simulink library "simetran"  (R2024b)
settings: Solver=VariableStepAuto  StartTime=0.0  StopTime=10.0  RelTol=1e-3
undefined symbols (not defined in the file): Csnu, gcbh, h, ResistanceM, Rsnu, Rt4, sps_rtmsupport, Ti, Ts, Z, Zm
libraries: fl_lib x81, nesl_utility x48, ee_lib x23
(part 1 of 3)
settings Model: Creator=Kyle  LastModifiedBy=CD8435

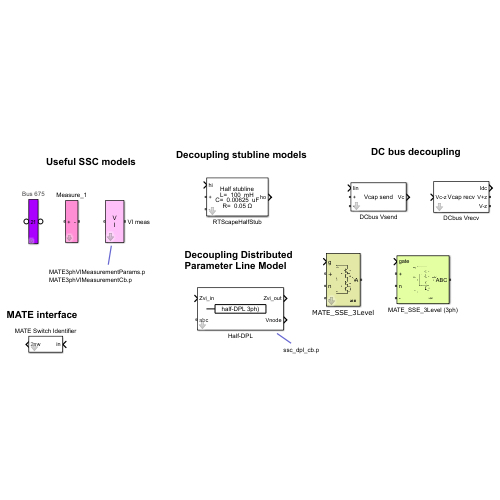
[thumbnail: Simulink's stored preview of the top-level diagram]
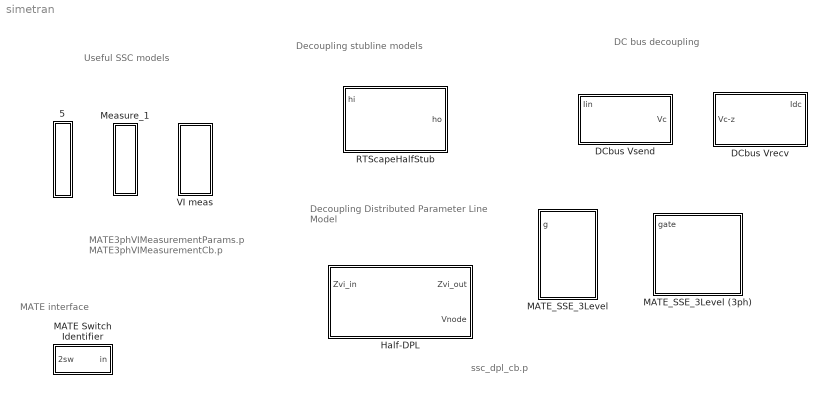
== system simetran ==
  note: ssc_dpl_cb.p
  note: MATE3phVIMeasurementParams.p
      | MATE3phVIMeasurementCb.p
  note: Decoupling stubline models
  note: Useful SSC models
  note: MATE interface
  note: DC bus decoupling
  note: Decoupling Distributed
      | Parameter Line Model
  5 : Subsystem  mask(Simscape Electrical Bus Numbering){bn=675}
      mask prompts: bn "Bus number"
      mask help: This block is a simple passthrough
      settings: AttributesFormatString=Bus %<bn>
  DCbus Vrecv : Subsystem  mask(DC Bus decoupling (Receiving-V)){Ts=Ts}
      mask prompts: Ts "Sample time (s)"
      mask help: This block is used to create a delay in DC-busses..
      mask Display: disp('Vcap recv')
  DCbus Vsend : Subsystem  mask(DC Bus decoupling (Sending-V)){Ts=Ts}
      mask prompts: Ts "Sample time (s)"
      mask help: This block is used to create a delay in DC-busses.
      mask Display: disp('Vcap send')
  Half-DPL : Subsystem  mask(Simscape 3-phase Distributed Parameters Line){Phases=3, Frequency=60, Resistance=[0.01273*2 0.3864], Inductance=[0.9337e-3  4.1264e-3], Capacitance=[12.74e-9 7.751e-9], Length=75, Ts=Ts}
      mask prompts: Phases "Number of phases N"; Frequency "Frequency used for R L C specification (Hz)"; Resistance "Resistance per unit length (Ohms/km)   [N*N matrix] or [R1 R0 R0m]"; Inductance "Inductance per unit length (H/km) [N*N matrix ] or [L1 L0 L0m]"; Capacitance "Capacitance per unit length (F/km) [N*N matrix] or [C1 C0 C0m]"; Length "Line length (km)"; Ts "Sample time (s)"
      mask help:
      | Implements a 3-phases distributed parameter line (DPL) model.
      |
      | One can either specify complete [NxN] matrices or simply enter sequence parameters vectors: the  positive and zero sequence parameters for a two-phase or  three-phase transposed  line, plus the mutual zero-sequence for a  six-phase transposed  line  (2 coupled 3-phase lines).
      |
      | This DPL model allows the decoupling of computational tasks at each line ends.
      mask init:
      | % Get current block
      | currentBlock = gcb;
      | 
      | % Get electric variables
      | [Zm,R,v,Ti,to,Rt4,h,Zimp,Zmat,Yphase,ResistanceM] = ssc_dpl_cb(gcb,'funcky balls', Phases, Frequency, Resistance, Inductance, Capacitance, Length);
      | 
      | delay=floor(to/Ts);
      | remd=rem(to,Ts)/Ts;
      | 
      | mess=['SimScape \n\n\n' ' DPL 3-ph'];
      mask TypeOptions Phases: 1 | 2 | 3 | 4 | 5 | 6 | 8 | 9 | 10 | 12
      mask Display:
      | plot(0,0,100,100,[20,20,80,80,80,80,20,20,10],[50,40,40,50,50,61,61,50,50])
      | disp('half-DPL 3ph)')
      | %disp(mess)
  MATE Switch Identifier : Subsystem  mask(MATE Switch Identifier){bn=Circuit BreakerEXP, bns=Circuit BreakerEXP, rsw=on, tagro=[]}
      mask prompts: bn "Switch block name (no ' ')"; bns "saved blockname"; rsw "Reverse switch logic"; tagro "Goto Tag (read only)"
      mask help: This block is used to identify switch signals for MATE optimization
      mask Callback bn:
      | this=gcb;
      | bns_x=get_param(this,'bns');
      | bn_x=get_param(this,'bn');
      | if ~isequal(bns_x, bn_x)
      |     set_param(this,'bns',bn_x);
      |     str=tempname;
      |     str=strrep(str(end-20:end),'_','x');
      |     str=['a' str];
      |     set_param([this '/Goto'],'Gototag',str);
      | end
      | gt=get_param([this '/Goto'],'GotoTag');
      | set_param([this],'tagro',gt);
      mask DialogControl Control2 Prompt: Note: Simscape electric breaker in open (OFF) when gate=1)
      mask DialogControl Control3 Prompt: Note: by using revert logic, it becomes like SPS breaker
  MATE_SSE_3Level : Subsystem  DialogController=POWERSYS.PowerSysDialog  mask(MATE 3-level NPC inverter){Arms=1, SnubberResistance=Rsnu, SnubberCapacitance=Csnu, Device=IGBT / Diodes, Ron=1e-3, Vf=1, ihiz=999}
      mask prompts: Arms "Number of bridge arms:"; SnubberResistance "Snubber resistance Rs (Ohms)"; SnubberCapacitance "Snubber capacitance Cs (F)"; Device "Power Electronic device (IGBT, GTO,MOSFET are equivalent)"; Ron "Internal resistance Ron (Ohms)"; Vf "Forward Device voltage  (V)"; ihiz "High Impedance current tolerance"
      mask help:
      | MATE Three-Level Bridge
      |
      | This model implements a 3-level NPC inverter using a surrogate circuit.
      | The surrogate circuit has only 3 switches and associated RC snubber.
      | The 3 switches connects the output phase connection A to each of inputs of inverter(V+, N, V-) and are controlled using an algorithm that mimics the behavior of real 3-level NPC inverters.
      |
      | Parameters:
      |
      | Snubber resistance Rs (Ohms): Resistance of the RC-snubber.
      | Snubber capacitance Cs (F): Capacitance of the RC snubber.
      | Internal resistance Ron (Ohms): Conduction resistance of all switches.
      |
      | gate signal (size 4). Drive the 4 IGBTs from the + rail to neutral rail, to the - rail in this order.
      mask init:
      | X.p1= [39 39 23.8000];
      |     X.p2= [44 56 49.6000 56 52.8000 56 61 61];
      |     X.p3= [44 44 44 61 61];
      |     X.p4= [75 67 83 75 67 83 75 75];
      |     X.p5= [61 75 75];
      |     X.p6= [75 75 61];
      |     X.p7= 0;
      | 
      |     Y.p1= [71 28 28];
      |     Y.p2= [  39.2000   33.6000   32.8000   33.6000   40.8000   33.6000  30.0000   12.4000];
      |     Y.p3= [28 71 60 66.4000 90];
      |     Y.p4= [54 42 42 54 54 54 54 66];
      |     Y.p5= [24 24 42];
      |     Y.p6= [66 76 76];
      |     Y.p7= 0;
      mask TypeOptions Arms: 1
      mask TypeOptions Device: IGBT / Diodes
  MATE_SSE_3Level (3ph) : Subsystem
  Measure_1 : Subsystem  DialogController=POWERSYS.PowerSysDialog  StartFcn=sps_rtmsupport('StartFcn',gcbh);  StopFcn=sps_rtmsupport('StopFcn',gcbh);  mask(Three-Phase Measurement){Va=Vabc_633_ssc, Ia=Iabc_633_ssc}
      mask prompts: Va "Voltage signal label  (use a From block to collect this signal)"; Ia "Current signal label  (use a From block to collect this signal)"
      mask help:
      | Ideal three-phase voltage and current measurements.
      |
      | The block outputs the voltages and currents in volts and amperes at the corresponding From blocks
      mask init:
      | bloc = gcb;
      | 
      | Vtag=get_param(bloc,'Va');
      | Itag=get_param(bloc,'Ia');
      | 
      | set_param([bloc '/Vabc'],'GotoTag',[Vtag]);
      | set_param([bloc '/Iabc'],'GotoTag',[Itag]);
      settings: UndoDeleteFcn=sps_rtmsupport('UndoDeleteFcn',gcbh);
      settings: LibrarySourceBlock=|
      | sps_lib/Sensors and Measurements/Three-Phase
      | V-I Measurement
      mask Help: helpview(psbhelp)
  RTScapeHalfStub : Subsystem  mask(SimScape Stubline){Phases=2 with differential inputs, pu=off, L=100e-3, Lpu=0.03, R=0.05, Rpu=0.02, S_base=75e3, V_base=1000, F_base=60, Ts=Ts}
      mask prompts: Phases "Number of phases N"; pu "Per-Unit value specification"; L "Inductance (H)"; Lpu "Inductance (pu)"; R "Resistance (Ohms)"; Rpu "Resistance (pu)"; S_base "Nominal Power (VA)"; V_base "Nominal voltage (V"; F_base "Nominal frequency (Hz)"; Ts "Sample time (s)"
      mask help:
      | The simScape Stubline block implements a single distributed parameters transmission line model with exactly one time step propagation delay. It is optimized for real-time simulation.
      |
      | The SimScape Stubline block permits the decoupling of system equations of networks on both sides of the stubline.
      mask init:
      | currentBlock = gcb;
      | 
      | 
      | 
      | % if isempty(S_base*V_base*F_base*Ts) 
      | %     return
      | % end
      | 
      | % Calculate Per Units
      | 
      | I_base=S_base/V_base;
      | w_base=2*pi*F_base;
      | Z_base=V_base/I_base;
      | L_base=Z_base/w_base;
      | C_base=1/(Z_base*w_base);
      | if pu == 1
      |     L=Lpu*L_base;
      |     R=Rpu*Z_base;
      | end
      | C = (Ts)^2/L;
      | Cpu = C / C_base;
      | 
      | 
      | 
      | 
      | 
      | 
      | % Calculate internal variables
      | [C, Zm, Rt4, h, w1, Z] = stub_cb(currentBlock,'lick it', 1, L, R, Ts);
      mask Help: eval('fts2help(''stubline'');');
      mask TypeOptions Phases: 1 | 2 | 3 | 4 | 5 | 6 | 2 with differential inputs
      mask Callback pu:
      | % Set mask display
      | stub_cb(gcb,'maskinitialization',1);
      mask Display: disp(sprintf('Half stubline\nL=  %s  mH\nC=  %s  uF\nR=  %s \\Omega',num2str(L*1e3,4), num2str(C*1e6,4), num2str(R,4)),'texmode','on');
  VI meas : Subsystem  mask(SimScape Three-Phase VI Measurement){VoltageMeasurement=phase-to-ground, SetLabelV=on, LabelV=Vabc_B1ssc, Vpu=on, VpuLL=off, CurrentMeasurement=yes, SetLabelI=on, LabelI=Iabc_B1ssc, Ipu=on, Pbase=100e6, Vbase=500e3}
      mask prompts: VoltageMeasurement "Voltage measurement"; SetLabelV "Use a label"; LabelV "Signal label  (use a From block to collect this signal)"; Vpu "Voltages in pu,  based on peak value of nominal phase-to-ground voltage"; VpuLL "Voltages in pu,  based on peak value of nominal phase-to-phase  voltage"; CurrentMeasurement "Current measurement"; SetLabelI "Use a label"; LabelI "Signal label  (use a From block to collect this signal)"; Ipu "Currents in pu"; Pbase "Base power ( VA 3 phase)"; Vbase "Nominal voltage used for pu measurement (Vrms phase-phase) :"
      mask help:
      | Three-phase voltage and current measurements.
      |
      | The block can output the voltages and currents in per unit values or in volts and amperes.
      mask init:
      | block = gcb;
      | Kv=1;
      | Ki=1;
      | 
      | [Kv ,Ki ]=MATE3phVIMeasurementParams(block ,Vpu ,VpuLL ,Ipu ,Vbase ,Pbase);
      | MATE3phVIMeasurementCb(block ,block);
      | 
      | 
      | vtype=get_param(block,'VoltageMeasurement');
      | if isequal(vtype,'phase-to-phase')
      |     str='ee.enum.vmeasurement.ll';
      | else
      |     str= 'ee.enum.vmeasurement.lg';
      | end
      | set_param([block '/Meas'],'vMeasurementType',str);
      mask TypeOptions VoltageMeasurement: no | phase-to-ground | phase-to-phase
      mask TypeOptions CurrentMeasurement: no | yes
      mask Display: disp(['V' 10 'I']);

== system simetran/5 ==
  Connection Port : PMIOPort  Side=Left
  Connection Port1 : PMIOPort  Port=2  Side=Right
  connections:
  Connection Port/RConn1 -- Connection Port1/RConn1

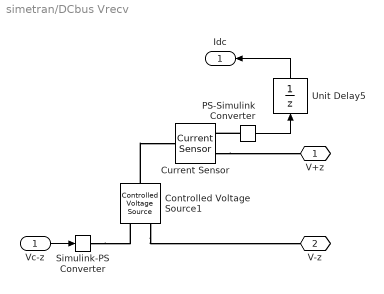
== system simetran/DCbus Vrecv ==
  Vc-z : Inport
  Controlled Voltage Source1 : fl_lib/Electrical/Electrical Sources/Controlled Voltage Source
  Current Sensor : fl_lib/Electrical/Electrical Sensors/Current Sensor
  PS-Simulink Converter : nesl_utility/PS-Simulink Converter  PhysicalDomain=network_engine_domain  SubClassName=ps_output  LeftPortType=input  RightPortType=output  PseudoPeriodic=off  Frequencies=[]  VectorFormat=inherit  Unit=inherit  AffineConversion=off
  Simulink-PS Converter : nesl_utility/Simulink-PS Converter  PhysicalDomain=network_engine_domain  SubClassName=ps_input  LeftPortType=input  RightPortType=output  PseudoPeriodic=off  Frequencies=[]  NoiseDistribution=none  NoiseParameters=[]  Unit=1  AffineConversion=off  FilteringAndDerivatives=provide  SimscapeFilterOrder=1  InputFilterTimeConstant=0.001  UdotUserProvided=0
  Unit Delay5 : UnitDelay  SampleTime=Ts  HasFrameUpgradeWarning=on
  V+z : PMIOPort  Side=Right
  V-z : PMIOPort  Port=2  Side=Right
  Idc : Outport
  wires:
  Vc-z/1 -> Simulink-PS Converter/1
  PS-Simulink Converter/1 -> Unit Delay5/1
  Unit Delay5/1 -> Idc/1
  connections:
  Controlled Voltage Source1/RConn2 -- V-z/RConn1
  Current Sensor/RConn2 -- V+z/RConn1
  PS-Simulink Converter/LConn1 -- Current Sensor/RConn1
  Controlled Voltage Source1/LConn1 -- Current Sensor/LConn1
  Simulink-PS Converter/RConn1 -- Controlled Voltage Source1/RConn1

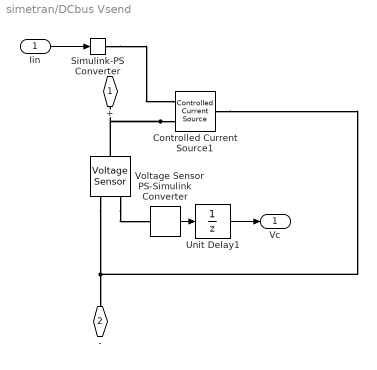
== system simetran/DCbus Vsend ==
  Iin : Inport
  Controlled Current Source1 : fl_lib/Electrical/Electrical Sources/Controlled Current Source
  PS-Simulink Converter : nesl_utility/PS-Simulink Converter  PhysicalDomain=network_engine_domain  SubClassName=ps_output  LeftPortType=input  RightPortType=output  PseudoPeriodic=off  Frequencies=[]  VectorFormat=1-D array  Unit=V  AffineConversion=off
  Simulink-PS Converter : nesl_utility/Simulink-PS Converter  PhysicalDomain=network_engine_domain  SubClassName=ps_input  LeftPortType=input  RightPortType=output  PseudoPeriodic=off  Frequencies=[]  NoiseDistribution=none  NoiseParameters=[]  Unit=1  AffineConversion=off  FilteringAndDerivatives=provide  SimscapeFilterOrder=1  InputFilterTimeConstant=0.001  UdotUserProvided=0
  Unit Delay1 : UnitDelay  SampleTime=Ts  HasFrameUpgradeWarning=on
  Voltage Sensor : fl_lib/Electrical/Electrical Sensors/Voltage Sensor
  + : PMIOPort  Side=Left
  - : PMIOPort  Port=2  Side=Left
  Vc : Outport
  wires:
  Iin/1 -> Simulink-PS Converter/1
  Unit Delay1/1 -> Vc/1
  PS-Simulink Converter/1 -> Unit Delay1/1
  connections:
  Simulink-PS Converter/RConn1 -- Controlled Current Source1/RConn1
  Controlled Current Source1/RConn2 -- Voltage Sensor/LConn1 -- +/RConn1
  Voltage Sensor/RConn1 -- PS-Simulink Converter/LConn1
  Controlled Current Source1/LConn1 -- Voltage Sensor/RConn2 -- -/RConn1

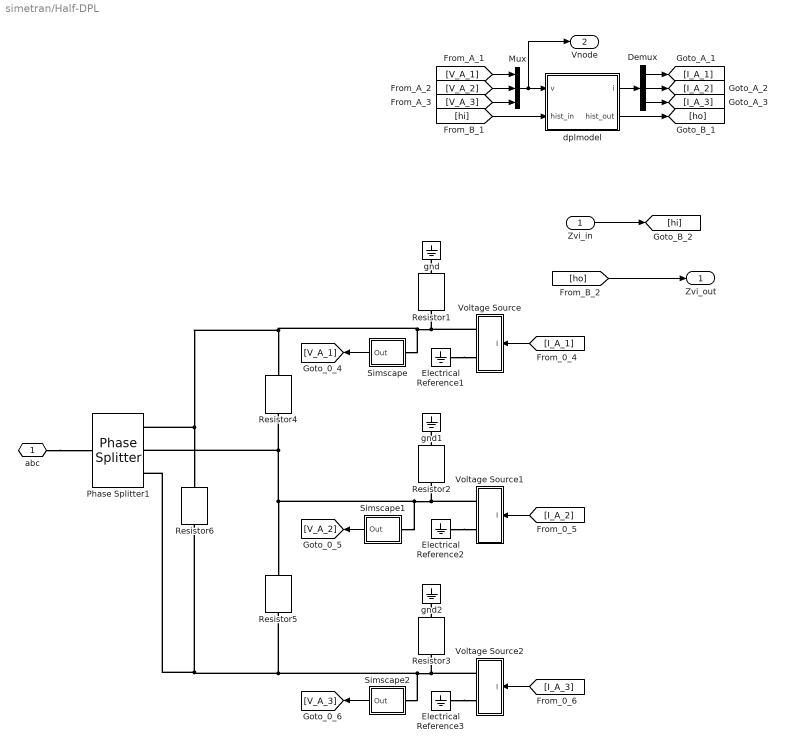
== system simetran/Half-DPL ==
  Zvi_in : Inport
  Demux : Demux  Outputs=3
      settings: DisplayOption=none
  Electrical Reference1 : fl_lib/Electrical/Electrical Elements/Electrical Reference
  Electrical Reference2 : fl_lib/Electrical/Electrical Elements/Electrical Reference
  Electrical Reference3 : fl_lib/Electrical/Electrical Elements/Electrical Reference
  Mux : Mux  Inputs=3
  Phase Splitter1 : ee_lib/Connectors & References/Phase Splitter
  Resistor1 : ee_lib/Passive/Resistor  R=ResistanceM(1,1) Ohm  enable_R_tol=ee.enum.toleranceApplication.none  R_tol=5  tol_distribution=ee.enum.toleranceDistribution.uniform  nSigma=4  enable_operating_limits=ee.enum.enable.no  operating_limit_action=ee.enum.passive.reportOpLim.warn  power_rating=1 W  max_working_voltage=100 V  noise_mode=ee.enum.sources.noise.Disabled  Tdevice=25 degC  sample_time=1e-3 s  repeatability=ee.enum.ic.repeatability.notRepeatable  user_seed=0  auto_seed=2758722926  fault_action=simscape.enum.assert.action.none  t_fault=1 s  power_derating_T1=70 degC  power_derating_T2=155 degC  operating_temperature_range_vec=[-50, 150] degC  alpha=3.93e-3 1/K  Tmeas=25 degC  thermal_mass=100 J/K  temperature_specify=off  temperature_priority=High  temperature=298.15 K  temperature_nominal_specify=off  temperature_nominal_value=1  temperature_nominal_unit=K
  Resistor2 : ee_lib/Passive/Resistor  R=ResistanceM(2,2) Ohm  enable_R_tol=ee.enum.toleranceApplication.none  R_tol=5  tol_distribution=ee.enum.toleranceDistribution.uniform  nSigma=4  enable_operating_limits=ee.enum.enable.no  operating_limit_action=ee.enum.passive.reportOpLim.warn  power_rating=1 W  max_working_voltage=100 V  noise_mode=ee.enum.sources.noise.Disabled  Tdevice=25 degC  sample_time=1e-3 s  repeatability=ee.enum.ic.repeatability.notRepeatable  user_seed=0  auto_seed=950329075  fault_action=simscape.enum.assert.action.none  t_fault=1 s  power_derating_T1=70 degC  power_derating_T2=155 degC  operating_temperature_range_vec=[-50, 150] degC  alpha=3.93e-3 1/K  Tmeas=25 degC  thermal_mass=100 J/K  temperature_specify=off  temperature_priority=High  temperature=298.15 K  temperature_nominal_specify=off  temperature_nominal_value=1  temperature_nominal_unit=K
  Resistor3 : ee_lib/Passive/Resistor  R=ResistanceM(3,3) Ohm  enable_R_tol=ee.enum.toleranceApplication.none  R_tol=5  tol_distribution=ee.enum.toleranceDistribution.uniform  nSigma=4  enable_operating_limits=ee.enum.enable.no  operating_limit_action=ee.enum.passive.reportOpLim.warn  power_rating=1 W  max_working_voltage=100 V  noise_mode=ee.enum.sources.noise.Disabled  Tdevice=25 degC  sample_time=1e-3 s  repeatability=ee.enum.ic.repeatability.notRepeatable  user_seed=0  auto_seed=3595130058  fault_action=simscape.enum.assert.action.none  t_fault=1 s  power_derating_T1=70 degC  power_derating_T2=155 degC  operating_temperature_range_vec=[-50, 150] degC  alpha=3.93e-3 1/K  Tmeas=25 degC  thermal_mass=100 J/K  temperature_specify=off  temperature_priority=High  temperature=298.15 K  temperature_nominal_specify=off  temperature_nominal_value=1  temperature_nominal_unit=K
  Resistor4 : ee_lib/Passive/Resistor  R=ResistanceM(1,2) Ohm  enable_R_tol=ee.enum.toleranceApplication.none  R_tol=5  tol_distribution=ee.enum.toleranceDistribution.uniform  nSigma=4  enable_operating_limits=ee.enum.enable.no  operating_limit_action=ee.enum.passive.reportOpLim.warn  power_rating=1 W  max_working_voltage=100 V  noise_mode=ee.enum.sources.noise.Disabled  Tdevice=25 degC  sample_time=1e-3 s  repeatability=ee.enum.ic.repeatability.notRepeatable  user_seed=0  auto_seed=4170736361  fault_action=simscape.enum.assert.action.none  t_fault=1 s  power_derating_T1=70 degC  power_derating_T2=155 degC  operating_temperature_range_vec=[-50, 150] degC  alpha=3.93e-3 1/K  Tmeas=25 degC  thermal_mass=100 J/K  temperature_specify=off  temperature_priority=High  temperature=298.15 K  temperature_nominal_specify=off  temperature_nominal_value=1  temperature_nominal_unit=K
  Resistor5 : ee_lib/Passive/Resistor  R=ResistanceM(2,3) Ohm  enable_R_tol=ee.enum.toleranceApplication.none  R_tol=5  tol_distribution=ee.enum.toleranceDistribution.uniform  nSigma=4  enable_operating_limits=ee.enum.enable.no  operating_limit_action=ee.enum.passive.reportOpLim.warn  power_rating=1 W  max_working_voltage=100 V  noise_mode=ee.enum.sources.noise.Disabled  Tdevice=25 degC  sample_time=1e-3 s  repeatability=ee.enum.ic.repeatability.notRepeatable  user_seed=0  auto_seed=3635143873  fault_action=simscape.enum.assert.action.none  t_fault=1 s  power_derating_T1=70 degC  power_derating_T2=155 degC  operating_temperature_range_vec=[-50, 150] degC  alpha=3.93e-3 1/K  Tmeas=25 degC  thermal_mass=100 J/K  temperature_specify=off  temperature_priority=High  temperature=298.15 K  temperature_nominal_specify=off  temperature_nominal_value=1  temperature_nominal_unit=K
  Resistor6 : ee_lib/Passive/Resistor  R=ResistanceM(1,3) Ohm  enable_R_tol=ee.enum.toleranceApplication.none  R_tol=5  tol_distribution=ee.enum.toleranceDistribution.uniform  nSigma=4  enable_operating_limits=ee.enum.enable.no  operating_limit_action=ee.enum.passive.reportOpLim.warn  power_rating=1 W  max_working_voltage=100 V  noise_mode=ee.enum.sources.noise.Disabled  Tdevice=25 degC  sample_time=1e-3 s  repeatability=ee.enum.ic.repeatability.notRepeatable  user_seed=0  auto_seed=2173251115  fault_action=simscape.enum.assert.action.none  t_fault=1 s  power_derating_T1=70 degC  power_derating_T2=155 degC  operating_temperature_range_vec=[-50, 150] degC  alpha=3.93e-3 1/K  Tmeas=25 degC  thermal_mass=100 J/K  temperature_specify=off  temperature_priority=High  temperature=298.15 K  temperature_nominal_specify=off  temperature_nominal_value=1  temperature_nominal_unit=K
  Simscape : Subsystem
      mask Display: disp('V')
  Simscape1 : Subsystem
      mask Display: disp('V')
  Simscape2 : Subsystem
      mask Display: disp('V')
  Voltage Source : Subsystem
  Voltage Source1 : Subsystem
  Voltage Source2 : Subsystem
  dplmodel : Subsystem
  gnd : fl_lib/Electrical/Electrical Elements/Electrical Reference
  gnd1 : fl_lib/Electrical/Electrical Elements/Electrical Reference
  gnd2 : fl_lib/Electrical/Electrical Elements/Electrical Reference
  abc : PMIOPort  Side=Left
  Zvi_out : Outport  VectorParamsAs1DForOutWhenUnconnected=off
  Vnode : Outport  Port=2  VectorParamsAs1DForOutWhenUnconnected=off
  wires:
  [I_A_1] -> Voltage Source/1(I)
  Simscape1/1(Out) -> [V_A_2]
  Simscape/1(Out) -> [V_A_1]
  [I_A_3] -> Voltage Source2/1(I)
  Simscape2/1(Out) -> [V_A_3]
  [I_A_2] -> Voltage Source1/1(I)
  dplmodel/2(hist_out) -> [ho]
  [hi] -> dplmodel/2(hist_in)
  Zvi_in/1 -> [hi]
  Mux/1 -> dplmodel/1(v), Vnode/1
  dplmodel/1(i) -> Demux/1
  [V_A_1] -> Mux/1
  Demux/1 -> [I_A_1]
  [V_A_2] -> Mux/2
  Demux/2 -> [I_A_2]
  [V_A_3] -> Mux/3
  Demux/3 -> [I_A_3]
  [ho] -> Zvi_out/1
  connections:
  abc/RConn1 -- Phase Splitter1/LConn1
  Resistor3/LConn1 -- gnd2/LConn1
  Electrical Reference1/LConn1 -- Voltage Source/RConn2
  Resistor2/LConn1 -- gnd1/LConn1
  Resistor1/LConn1 -- gnd/LConn1
  Electrical Reference3/LConn1 -- Voltage Source2/RConn2
  Electrical Reference2/LConn1 -- Voltage Source1/RConn2
  Phase Splitter1/RConn2 -- Resistor4/RConn1 -- Simscape1/LConn1 -- Voltage Source1/RConn1 -- Resistor2/RConn1 -- Resistor5/LConn1
  Phase Splitter1/RConn3 -- Resistor3/RConn1 -- Voltage Source2/RConn1 -- Simscape2/LConn1 -- Resistor5/RConn1 -- Resistor6/RConn1
  Phase Splitter1/RConn1 -- Resistor6/LConn1 -- Resistor4/LConn1 -- Resistor1/RConn1 -- Voltage Source/RConn1 -- Simscape/LConn1

== system simetran/MATE Switch Identifier ==
  in : Inport
  Constant : Constant  Value=rsw
  Switch : Switch  Criteria=u2 > Threshold  Threshold=0.5  SaturateOnIntegerOverflow=off  InputSameDT=off
  inv1 : Subsystem
  2sw : Outport
  tag scope: a58fxa8a9x743c756a9e3e=global
  wires:
  in/1 -> [a58fxa8a9x743c756a9e3e], Switch/3, inv1/1(gate)
  inv1/1(Out1) -> Switch/1
  Switch/1 -> 2sw/1
  Constant/1 -> Switch/2

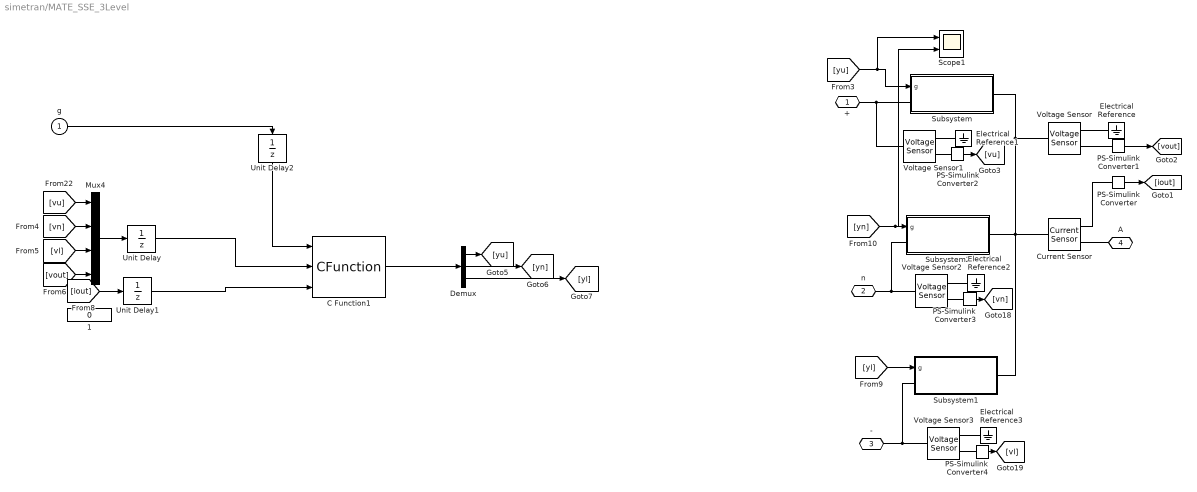
== system simetran/MATE_SSE_3Level ==
  g : Inport
  1 : Constant  Value=0
  C Function1 : CFunction  OutputCode=|  InitializeConditionsCode=status_old=0;  CodegenOutputCode=|  CodegenInitializeConditionsCode=status_old=0;  CustomCodeSettingLocation=ModelConfigurationParameters
      OutputCode=|
      | {
      |     double status;
      | 
      |     //InputRealPtrsType gg      = ssGetInputPortRealSignalPtrs(S,0);
      |     //InputRealPtrsType Vtermm  = ssGetInputPortRealSignalPtrs(S,1);
      |     //InputRealPtrsType ioutt   = ssGetInputPortRealSignalPtrs(S,2);
      |     //InputRealPtrsType tol     = ssGetInputPortRealSignalPtrs(S,3);
      | 
      | 
      |     //real_T            *sw       =  ssGetOutputPortRealSignal(S,0);  // sw
      |     //real_T			  *stat     =  ssGetOutputPortRealSignal(S,1);  // status
      | 
      | 
      | 
      |     //mexPrintf("OUTPUTpause:\n");
      |     //mexEvalString("pause(2);");
      | 
      | 
      | 
      |     //real_T *status_old    = (real_T*) ssGetDWork(S,0);
      |     //real_T status[1];
      | 
      | 
      |     //real_T  g[4];
      |     //real_T  Vterm[4];
      |  
      | 
      |     //real_T iout[1];
      | 
      |    // *(g+0)= *gg[0];
      |    // *(g+1)= *gg[1];
      |    // *(g+2)= *gg[2];
      |    // *(g+3)= *gg[3];
      | 
      |    // *(Vterm+0)= *Vtermm[0];
      |    // *(Vterm+1)= *Vtermm[1];
      |    // *(Vterm+2)= *Vtermm[2];
      |    // *(Vterm+3)= *Vtermm[3];
      | 
      |    // iout= *ioutt[0];
      | 
      | 
      |  
      | 
      | 
      |     if (*(g+0)>0.5 && *(g+1)>0.5) {
      |         *(sw+0)=1;*(sw+1)=0;*(sw+2)=0;status=1;
      |     }
      |     else if (*(g+2)>0.5  && *(g+3)>0.5) {
      |         *(sw+0)=0;*(sw+1)=0;*(sw+2)=1;status=2;
      |     }
      |     else if (*(g+1)>0.5  && *(g+2)>0.5) {
      |         *(sw+0)=0;*(sw+1)=1;*(sw+2)=0;status=3;
      |     }
      |     else if (*(g+1)>0.5 && iout>0) {
      |         *(sw+0)=0;*(sw+1)=1;*(sw+2)=0;status=4;
      |     }
      |     else if (*(g+2)>0.5 && iout<0) {
      |         *(sw+0)=0;*(sw+1)=1;*(sw+2)=0;status=5;
      |     }
      |     else if ( (iout>0 && status_old<=6)) { //|| (*(iout>tol[0] && status_old>5) )  {
      |         *(sw+0)=0;*(sw+1)=0;*(sw+2)=1;status=6;
      |     }
      |     else if ( (iout<0 && status_old<=5) || (iout<0 && status_old==7) ) { // || (iout<(0-tol[0]) && status_old[0]>5)   ) {
      |         *(sw+0)=1;*(sw+1)=0;*(sw+2)=0;status=7;
      |     }
      |     else if ( (*(Vterm+3)>*(Vterm+1) && *(g+2)>0.5) || (*(Vterm+3)<*(Vterm+1)  && *(g+1)>0.5) ) {
      |         *(sw+0)=0;*(sw+1)=1;*(sw+2)=0;status=8;
      |     }
      |     else if (*(Vterm+3)>*(Vterm+0)) {
      |         *(sw+0)=1;*(sw+1)=0;*(sw+2)=0;status=9;
      |     }
      |     else if (*(Vterm+3)<*(Vterm+2)) {
      |         *(sw+0)=0;*(sw+1)=0;*(sw+2)=1;status=10;
      |     }
      |     else {
      |         *(sw+0)=0;*(sw+1)=0;*(sw+2)=0;status=11;
      |     }
      | 
      | 
      | 
      |     status_old=status;
      | 
      | 
      | }
      CodegenOutputCode=|
      | {
      |     double status;
      | 
      |     //InputRealPtrsType gg      = ssGetInputPortRealSignalPtrs(S,0);
      |     //InputRealPtrsType Vtermm  = ssGetInputPortRealSignalPtrs(S,1);
      |     //InputRealPtrsType ioutt   = ssGetInputPortRealSignalPtrs(S,2);
      |     //InputRealPtrsType tol     = ssGetInputPortRealSignalPtrs(S,3);
      | 
      | 
      |     //real_T            *sw       =  ssGetOutputPortRealSignal(S,0);  // sw
      |     //real_T			  *stat     =  ssGetOutputPortRealSignal(S,1);  // status
      | 
      | 
      | 
      |     //mexPrintf("OUTPUTpause:\n");
      |     //mexEvalString("pause(2);");
      | 
      | 
      | 
      |     //real_T *status_old    = (real_T*) ssGetDWork(S,0);
      |     //real_T status[1];
      | 
      | 
      |     //real_T  g[4];
      |     //real_T  Vterm[4];
      |  
      | 
      |     //real_T iout[1];
      | 
      |    // *(g+0)= *gg[0];
      |    // *(g+1)= *gg[1];
      |    // *(g+2)= *gg[2];
      |    // *(g+3)= *gg[3];
      | 
      |    // *(Vterm+0)= *Vtermm[0];
      |    // *(Vterm+1)= *Vtermm[1];
      |    // *(Vterm+2)= *Vtermm[2];
      |    // *(Vterm+3)= *Vtermm[3];
      | 
      |    // iout= *ioutt[0];
      | 
      | 
      |  
      | 
      | 
      |     if (*(g+0)>0.5 && *(g+1)>0.5) {
      |         *(sw+0)=1;*(sw+1)=0;*(sw+2)=0;status=1;
      |     }
      |     else if (*(g+2)>0.5  && *(g+3)>0.5) {
      |         *(sw+0)=0;*(sw+1)=0;*(sw+2)=1;status=2;
      |     }
      |     else if (*(g+1)>0.5  && *(g+2)>0.5) {
      |         *(sw+0)=0;*(sw+1)=1;*(sw+2)=0;status=3;
      |     }
      |     else if (*(g+1)>0.5 && iout>0) {
      |         *(sw+0)=0;*(sw+1)=1;*(sw+2)=0;status=4;
      |     }
      |     else if (*(g+2)>0.5 && iout<0) {
      |         *(sw+0)=0;*(sw+1)=1;*(sw+2)=0;status=5;
      |     }
      |     else if ( (iout>0 && status_old<=6)) { //|| (*(iout>tol[0] && status_old>5) )  {
      |         *(sw+0)=0;*(sw+1)=0;*(sw+2)=1;status=6;
      |     }
      |     else if ( (iout<0 && status_old<=5) || (iout<0 && status_old==7) ) { // || (iout<(0-tol[0]) && status_old[0]>5)   ) {
      |         *(sw+0)=1;*(sw+1)=0;*(sw+2)=0;status=7;
      |     }
      |     else if ( (*(Vterm+3)>*(Vterm+1) && *(g+2)>0.5) || (*(Vterm+3)<*(Vterm+1)  && *(g+1)>0.5) ) {
      |         *(sw+0)=0;*(sw+1)=1;*(sw+2)=0;status=8;
      |     }
      |     else if (*(Vterm+3)>*(Vterm+0)) {
      |         *(sw+0)=1;*(sw+1)=0;*(sw+2)=0;status=9;
      |     }
      |     else if (*(Vterm+3)<*(Vterm+2)) {
      |         *(sw+0)=0;*(sw+1)=0;*(sw+2)=1;status=10;
      |     }
      |     else {
      |         *(sw+0)=0;*(sw+1)=0;*(sw+2)=0;status=11;
      |     }
      | 
      | 
      | 
      |     status_old=status;
      | 
      | 
      | }
  Current Sensor : fl_lib/Electrical/Electrical Sensors/Current Sensor
  Demux : Demux  Outputs=3
  Electrical Reference{,1..3} (4 alike) : fl_lib/Electrical/Electrical Elements/Electrical Reference
  Mux4 : Mux
  PS-Simulink Converter{,1..4} (5 alike) : nesl_utility/PS-Simulink Converter  PhysicalDomain=network_engine_domain  SubClassName=ps_output  LeftPortType=input  RightPortType=output  PseudoPeriodic=off  Frequencies=[]  VectorFormat=inherit  Unit=inherit  AffineConversion=off
  Scope1 : Scope  NumInputPorts=2
  Subsystem : Subsystem
  Subsystem1 : Subsystem
  Subsystem2 : Subsystem
  Unit Delay : UnitDelay  SampleTime=Ts  HasFrameUpgradeWarning=on
  Unit Delay1 : UnitDelay  SampleTime=Ts  HasFrameUpgradeWarning=on
  Unit Delay2 : UnitDelay  SampleTime=Ts  HasFrameUpgradeWarning=on
  Voltage Sensor{,1..3} (4 alike) : fl_lib/Electrical/Electrical Sensors/Voltage Sensor
  + : PMIOPort  Side=Left
  n : PMIOPort  Port=2  Side=Left
  - : PMIOPort  Port=3  Side=Left
  A : PMIOPort  Port=4  Side=Right
  wires:
  Mux4/1 -> Unit Delay/1
  Demux/2 -> [yn]
  [vu] -> Mux4/1
  [vn] -> Mux4/2
  [vl] -> Mux4/3
  [vout] -> Mux4/4
  g/1 -> Unit Delay2/1
  Demux/3 -> [yl]
  Demux/1 -> [yu]
  [yu] -> Scope1/1, Subsystem/1(g)
  [yl] -> Subsystem1/1(g)
  [yn] -> Subsystem2/1(g), Scope1/2
  PS-Simulink Converter/1 -> [iout]
  PS-Simulink Converter1/1 -> [vout]
  PS-Simulink Converter2/1 -> [vu]
  PS-Simulink Converter3/1 -> [vn]
  PS-Simulink Converter4/1 -> [vl]
  [iout] -> Unit Delay1/1
  C Function1/1 -> Demux/1
  Unit Delay/1 -> C Function1/2
  Unit Delay1/1 -> C Function1/3
  Unit Delay2/1 -> C Function1/1
  connections:
  +/RConn1 -- Subsystem/LConn1 -- Voltage Sensor1/LConn1
  -/RConn1 -- Subsystem1/LConn1 -- Voltage Sensor3/LConn1
  Current Sensor/LConn1 -- Subsystem1/RConn1 -- Subsystem2/RConn1 -- Subsystem/RConn1 -- Voltage Sensor/LConn1
  n/RConn1 -- Subsystem2/LConn1 -- Voltage Sensor2/LConn1
  A/RConn1 -- Current Sensor/RConn2
  PS-Simulink Converter/LConn1 -- Current Sensor/RConn1
  Voltage Sensor/RConn2 -- Electrical Reference/LConn1
  Voltage Sensor/RConn1 -- PS-Simulink Converter1/LConn1
  Voltage Sensor1/RConn2 -- Electrical Reference1/LConn1
  Voltage Sensor1/RConn1 -- PS-Simulink Converter2/LConn1
  Voltage Sensor2/RConn1 -- PS-Simulink Converter3/LConn1
  Voltage Sensor2/RConn2 -- Electrical Reference2/LConn1
  Voltage Sensor3/RConn2 -- Electrical Reference3/LConn1
  Voltage Sensor3/RConn1 -- PS-Simulink Converter4/LConn1

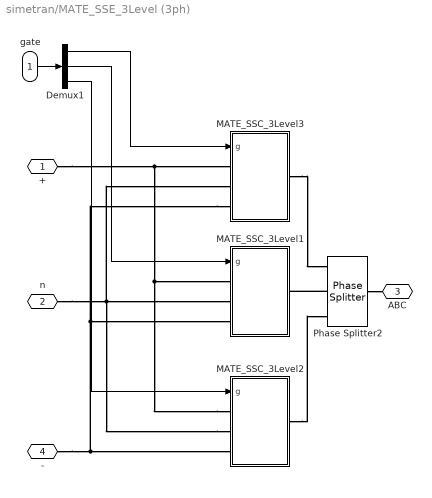
== system simetran/MATE_SSE_3Level (3ph) ==
  gate : Inport
  Demux1 : Demux  Outputs=[4 4 4]
  MATE_SSC_3Level1 : Subsystem  DialogController=POWERSYS.PowerSysDialog  mask(MATE 3-level NPC inverter){Arms=1, SnubberResistance=Rsnu, SnubberCapacitance=Csnu, Device=IGBT / Diodes, Ron=1e-3, Vf=1, ihiz=999}
      mask prompts: Arms "Number of bridge arms:"; SnubberResistance "Snubber resistance Rs (Ohms)"; SnubberCapacitance "Snubber capacitance Cs (F)"; Device "Power Electronic device (IGBT, GTO,MOSFET are equivalent)"; Ron "Internal resistance Ron (Ohms)"; Vf "Forward Device voltage  (V)"; ihiz "High Impedance current tolerance"
      mask help:
      | MATE Three-Level Bridge
      |
      | This model implements a 3-level NPC inverter using a surrogate circuit.
      | The surrogate circuit has only 3 switches and associated RC snubber.
      | The 3 switches connects the output phase connection A to each of inputs of inverter(V+, N, V-) and are controlled using an algorithm that mimics the behavior of real 3-level NPC inverters.
      |
      | Parameters:
      |
      | Snubber resistance Rs (Ohms): Resistance of the RC-snubber.
      | Snubber capacitance Cs (F): Capacitance of the RC snubber.
      | Internal resistance Ron (Ohms): Conduction resistance of all switches.
      |
      | gate signal (size 4). Drive the 4 IGBTs from the + rail to neutral rail, to the - rail in this order.
      mask init: same as simetran/MATE_SSE_3Level
      mask TypeOptions Arms: 1
      mask TypeOptions Device: IGBT / Diodes
  MATE_SSC_3Level2 : Subsystem  DialogController=POWERSYS.PowerSysDialog  mask(MATE 3-level NPC inverter){Arms=1, SnubberResistance=Rsnu, SnubberCapacitance=Csnu, Device=IGBT / Diodes, Ron=1e-3, Vf=1, ihiz=999}
      mask prompts: Arms "Number of bridge arms:"; SnubberResistance "Snubber resistance Rs (Ohms)"; SnubberCapacitance "Snubber capacitance Cs (F)"; Device "Power Electronic device (IGBT, GTO,MOSFET are equivalent)"; Ron "Internal resistance Ron (Ohms)"; Vf "Forward Device voltage  (V)"; ihiz "High Impedance current tolerance"
      mask help:
      | MATE Three-Level Bridge
      |
      | This model implements a 3-level NPC inverter using a surrogate circuit.
      | The surrogate circuit has only 3 switches and associated RC snubber.
      | The 3 switches connects the output phase connection A to each of inputs of inverter(V+, N, V-) and are controlled using an algorithm that mimics the behavior of real 3-level NPC inverters.
      |
      | Parameters:
      |
      | Snubber resistance Rs (Ohms): Resistance of the RC-snubber.
      | Snubber capacitance Cs (F): Capacitance of the RC snubber.
      | Internal resistance Ron (Ohms): Conduction resistance of all switches.
      |
      | gate signal (size 4). Drive the 4 IGBTs from the + rail to neutral rail, to the - rail in this order.
      mask init: same as simetran/MATE_SSE_3Level
      mask TypeOptions Arms: 1
      mask TypeOptions Device: IGBT / Diodes
  MATE_SSC_3Level3 : Subsystem  DialogController=POWERSYS.PowerSysDialog  mask(MATE 3-level NPC inverter){Arms=1, SnubberResistance=Rsnu, SnubberCapacitance=Csnu, Device=IGBT / Diodes, Ron=1e-3, Vf=1, ihiz=999}
      mask prompts: Arms "Number of bridge arms:"; SnubberResistance "Snubber resistance Rs (Ohms)"; SnubberCapacitance "Snubber capacitance Cs (F)"; Device "Power Electronic device (IGBT, GTO,MOSFET are equivalent)"; Ron "Internal resistance Ron (Ohms)"; Vf "Forward Device voltage  (V)"; ihiz "High Impedance current tolerance"
      mask help:
      | MATE Three-Level Bridge
      |
      | This model implements a 3-level NPC inverter using a surrogate circuit.
      | The surrogate circuit has only 3 switches and associated RC snubber.
      | The 3 switches connects the output phase connection A to each of inputs of inverter(V+, N, V-) and are controlled using an algorithm that mimics the behavior of real 3-level NPC inverters.
      |
      | Parameters:
      |
      | Snubber resistance Rs (Ohms): Resistance of the RC-snubber.
      | Snubber capacitance Cs (F): Capacitance of the RC snubber.
      | Internal resistance Ron (Ohms): Conduction resistance of all switches.
      |
      | gate signal (size 4). Drive the 4 IGBTs from the + rail to neutral rail, to the - rail in this order.
      mask init: same as simetran/MATE_SSE_3Level
      mask TypeOptions Arms: 1
      mask TypeOptions Device: IGBT / Diodes
  Phase Splitter2 : ee_lib/Connectors & References/Phase Splitter
  + : PMIOPort  Side=Left
  n : PMIOPort  Port=2  Side=Left
  ABC : PMIOPort  Port=3  Side=Right
  - : PMIOPort  Port=4  Side=Left
  wires:
  Demux1/3 -> MATE_SSC_3Level2/1(g)
  Demux1/2 -> MATE_SSC_3Level1/1(g)
  Demux1/1 -> MATE_SSC_3Level3/1(g)
  gate/1 -> Demux1/1
  connections:
  MATE_SSC_3Level2/RConn1 -- Phase Splitter2/RConn3
  MATE_SSC_3Level3/RConn1 -- Phase Splitter2/RConn1
  Phase Splitter2/RConn2 -- MATE_SSC_3Level1/RConn1
  Phase Splitter2/LConn1 -- ABC/RConn1
  MATE_SSC_3Level3/LConn3 -- MATE_SSC_3Level1/LConn3 -- -/RConn1 -- MATE_SSC_3Level2/LConn3
  MATE_SSC_3Level2/LConn2 -- MATE_SSC_3Level1/LConn2 -- n/RConn1 -- MATE_SSC_3Level3/LConn2
  MATE_SSC_3Level2/LConn1 -- MATE_SSC_3Level1/LConn1 -- +/RConn1 -- MATE_SSC_3Level3/LConn1

== system simetran/Measure_1 ==
  Current and Voltage Sensor (Three-Phase) : ee_lib/Sensors & Transducers/Current and Voltage Sensor (Three-Phase)  vMeasurementType=ee.enum.vmeasurement.ll  outputUnit=ee.enum.unit.si  SRated=100e6 A*V  VRated=24e3 V  I_specify=off  I_priority=None  I=[0, 0, 0] A  I_nominal_specify=off  I_nominal_value=1  I_nominal_unit=A  V_specify=off  V_priority=None  V=[0, 0, 0] V  V_nominal_specify=off  V_nominal_value=1  V_nominal_unit=V
      settings: InternalSimscapePortConfiguration="{\"Bottom\":[],\"Left\":[{\"id\":\"N1\",\"label\":\"~1\",\"type\":\"foundation.electrical.three_phase\"}],\"Right\":[{\"id\":\"V_output\",\"label\":\"V\",\"type\":\"output\"},{\"id\":\"I_output\",\"label\":\"I\",\"type\":\"output\"},{\"id\":\"N2\",\"label\":\"~2\",\"type\":\"foundation.electrical.three_phase\"}],\"Top\":[]}"
  PS-Simulink Converter : nesl_utility/PS-Simulink Converter  PhysicalDomain=network_engine_domain  SubClassName=ps_output  LeftPortType=input  RightPortType=output  PseudoPeriodic=off  Frequencies=[]  VectorFormat=inherit  Unit=inherit  AffineConversion=off
  PS-Simulink Converter1 : nesl_utility/PS-Simulink Converter  PhysicalDomain=network_engine_domain  SubClassName=ps_output  LeftPortType=input  RightPortType=output  PseudoPeriodic=off  Frequencies=[]  VectorFormat=inherit  Unit=inherit  AffineConversion=off
  + : PMIOPort  Side=Left
  - : PMIOPort  Port=2  Side=Right
  tag scope: Iabc_633_ssc=global, Vabc_633_ssc=global
  wires:
  PS-Simulink Converter/1 -> [Vabc_633_ssc]
  PS-Simulink Converter1/1 -> [Iabc_633_ssc]
  connections:
  Current and Voltage Sensor (Three-Phase)/RConn2 -- PS-Simulink Converter1/LConn1
  Current and Voltage Sensor (Three-Phase)/RConn1 -- PS-Simulink Converter/LConn1
  Current and Voltage Sensor (Three-Phase)/LConn1 -- +/RConn1
  Current and Voltage Sensor (Three-Phase)/RConn3 -- -/RConn1

== system simetran/RTScapeHalfStub ==
  hi : Inport
  SL1 : Subsystem
      mask Display: disp('stubline');
  + : PMIOPort  Side=Left
  - : PMIOPort  Port=2  Side=Left
  ho : Outport  VectorParamsAs1DForOutWhenUnconnected=off
  wires:
  SL1/1(o) -> ho/1
  hi/1 -> SL1/1(i)
  connections:
  +/RConn1 -- SL1/LConn1
  -/RConn1 -- SL1/RConn1

== system simetran/VI meas ==
  Kv2 : Gain  Gain=Kv  SaturateOnIntegerOverflow=on  OutDataTypeStr=Inherit: Same as input  ParamDataTypeStr=Inherit: Same as input
  Kv3 : Gain  Gain=Ki  SaturateOnIntegerOverflow=on  OutDataTypeStr=Inherit: Same as input  ParamDataTypeStr=Inherit: Same as input
  Meas : ee_lib/Sensors & Transducers/Current and Voltage Sensor (Three-Phase)  vMeasurementType=ee.enum.vmeasurement.lg  outputUnit=ee.enum.unit.si  SRated=100e6 A*V  VRated=24e3 V  I_specify=off  I_priority=None  I=[0, 0, 0] A  I_nominal_specify=off  I_nominal_value=1  I_nominal_unit=A  V_specify=off  V_priority=None  V=[0, 0, 0] V  V_nominal_specify=off  V_nominal_value=1  V_nominal_unit=V
      settings: InternalSimscapePortConfiguration="{\"Bottom\":[],\"Left\":[{\"id\":\"N1\",\"label\":\"~1\",\"type\":\"foundation.electrical.three_phase\"}],\"Right\":[{\"id\":\"V_output\",\"label\":\"V\",\"type\":\"output\"},{\"id\":\"I_output\",\"label\":\"I\",\"type\":\"output\"},{\"id\":\"N2\",\"label\":\"~2\",\"type\":\"foundation.electrical.three_phase\"}],\"Top\":[]}"
  PS-Simulink Converter : nesl_utility/PS-Simulink Converter  PhysicalDomain=network_engine_domain  SubClassName=ps_output  LeftPortType=input  RightPortType=output  PseudoPeriodic=off  Frequencies=[]  VectorFormat=inherit  Unit=inherit  AffineConversion=off
  PS-Simulink Converter1 : nesl_utility/PS-Simulink Converter  PhysicalDomain=network_engine_domain  SubClassName=ps_output  LeftPortType=input  RightPortType=output  PseudoPeriodic=off  Frequencies=[]  VectorFormat=inherit  Unit=inherit  AffineConversion=off
  + : PMIOPort  Side=Left
  - : PMIOPort  Port=2  Side=Right
  tag scope: Iabc_B1ssc=global, Vabc_B1ssc=global
  wires:
  Kv3/1 -> [Iabc_B1ssc]
  Kv2/1 -> [Vabc_B1ssc]
  PS-Simulink Converter1/1 -> Kv3/1
  PS-Simulink Converter/1 -> Kv2/1
  connections:
  Meas/RConn1 -- PS-Simulink Converter/LConn1
  Meas/LConn1 -- +/RConn1
  Meas/RConn2 -- PS-Simulink Converter1/LConn1
  Meas/RConn3 -- -/RConn1

== system simetran/Half-DPL/Simscape ==
  Electrical Reference1 : fl_lib/Electrical/Electrical Elements/Electrical Reference
  PS-S : nesl_utility/PS-Simulink Converter  PhysicalDomain=network_engine_domain  SubClassName=ps_output  LeftPortType=input  RightPortType=output  PseudoPeriodic=off  Frequencies=[]  VectorFormat=1-D array  Unit=V  AffineConversion=off
  Voltage Sensor : fl_lib/Electrical/Electrical Sensors/Voltage Sensor
  V : PMIOPort  Side=Left
  Out : Outport  VectorParamsAs1DForOutWhenUnconnected=off
  wires:
  PS-S/1 -> Out/1  "voltage"
  connections:
  PS-S/LConn1 -- Voltage Sensor/RConn1
  V/RConn1 -- Voltage Sensor/LConn1
  Electrical Reference1/LConn1 -- Voltage Sensor/RConn2

== system simetran/Half-DPL/Simscape1 ==
  Electrical Reference1 : fl_lib/Electrical/Electrical Elements/Electrical Reference
  PS-S : nesl_utility/PS-Simulink Converter  PhysicalDomain=network_engine_domain  SubClassName=ps_output  LeftPortType=input  RightPortType=output  PseudoPeriodic=off  Frequencies=[]  VectorFormat=1-D array  Unit=V  AffineConversion=off
  Voltage Sensor : fl_lib/Electrical/Electrical Sensors/Voltage Sensor
  V : PMIOPort  Side=Left
  Out : Outport  VectorParamsAs1DForOutWhenUnconnected=off
  wires:
  PS-S/1 -> Out/1  "voltage"
  connections:
  Electrical Reference1/LConn1 -- Voltage Sensor/RConn2
  V/RConn1 -- Voltage Sensor/LConn1
  PS-S/LConn1 -- Voltage Sensor/RConn1

== system simetran/Half-DPL/Simscape2 ==
  Electrical Reference1 : fl_lib/Electrical/Electrical Elements/Electrical Reference
  PS-S : nesl_utility/PS-Simulink Converter  PhysicalDomain=network_engine_domain  SubClassName=ps_output  LeftPortType=input  RightPortType=output  PseudoPeriodic=off  Frequencies=[]  VectorFormat=1-D array  Unit=V  AffineConversion=off
  Voltage Sensor : fl_lib/Electrical/Electrical Sensors/Voltage Sensor
  V : PMIOPort  Side=Left
  Out : Outport  VectorParamsAs1DForOutWhenUnconnected=off
  wires:
  PS-S/1 -> Out/1  "voltage"
  connections:
  PS-S/LConn1 -- Voltage Sensor/RConn1
  V/RConn1 -- Voltage Sensor/LConn1
  Electrical Reference1/LConn1 -- Voltage Sensor/RConn2

== system simetran/Half-DPL/Voltage Source ==
  I : Inport
  Controlled Current Source1 : fl_lib/Electrical/Electrical Sources/Controlled Current Source
  Simulink-PS Converter : nesl_utility/Simulink-PS Converter  PhysicalDomain=network_engine_domain  SubClassName=ps_input  LeftPortType=input  RightPortType=output  PseudoPeriodic=off  Frequencies=[]  NoiseDistribution=none  NoiseParameters=[]  Unit=1  AffineConversion=off  FilteringAndDerivatives=zero  SimscapeFilterOrder=1  InputFilterTimeConstant=.001  UdotUserProvided=0
  + : PMIOPort  Side=Right
  - : PMIOPort  Port=2  Side=Right
  wires:
  I/1 -> Simulink-PS Converter/1
  connections:
  Controlled Current Source1/RConn1 -- Simulink-PS Converter/RConn1
  Controlled Current Source1/RConn2 -- -/RConn1
  Controlled Current Source1/LConn1 -- +/RConn1

== system simetran/Half-DPL/Voltage Source1 ==
  I : Inport
  Controlled Current Source1 : fl_lib/Electrical/Electrical Sources/Controlled Current Source
  Simulink-PS Converter : nesl_utility/Simulink-PS Converter  PhysicalDomain=network_engine_domain  SubClassName=ps_input  LeftPortType=input  RightPortType=output  PseudoPeriodic=off  Frequencies=[]  NoiseDistribution=none  NoiseParameters=[]  Unit=1  AffineConversion=off  FilteringAndDerivatives=zero  SimscapeFilterOrder=1  InputFilterTimeConstant=.001  UdotUserProvided=0
  + : PMIOPort  Side=Right
  - : PMIOPort  Port=2  Side=Right
  wires:
  I/1 -> Simulink-PS Converter/1
  connections:
  Controlled Current Source1/LConn1 -- +/RConn1
  Controlled Current Source1/RConn2 -- -/RConn1
  Controlled Current Source1/RConn1 -- Simulink-PS Converter/RConn1

== system simetran/Half-DPL/Voltage Source2 ==
  I : Inport
  Controlled Current Source1 : fl_lib/Electrical/Electrical Sources/Controlled Current Source
  Simulink-PS Converter : nesl_utility/Simulink-PS Converter  PhysicalDomain=network_engine_domain  SubClassName=ps_input  LeftPortType=input  RightPortType=output  PseudoPeriodic=off  Frequencies=[]  NoiseDistribution=none  NoiseParameters=[]  Unit=1  AffineConversion=off  FilteringAndDerivatives=zero  SimscapeFilterOrder=1  InputFilterTimeConstant=.001  UdotUserProvided=0
  + : PMIOPort  Side=Right
  - : PMIOPort  Port=2  Side=Right
  wires:
  I/1 -> Simulink-PS Converter/1
  connections:
  Controlled Current Source1/RConn1 -- Simulink-PS Converter/RConn1
  Controlled Current Source1/RConn2 -- -/RConn1
  Controlled Current Source1/LConn1 -- +/RConn1

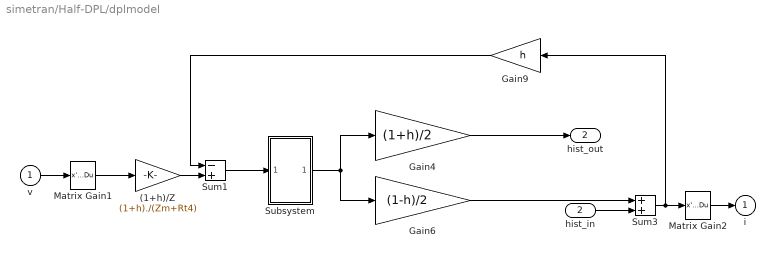
== system simetran/Half-DPL/dplmodel ==
  v : Inport
  hist_in : Inport  Port=2
  (1+h)/Z : Gain  Gain=(1+h)./(Zm+Rt4)  SaturateOnIntegerOverflow=on  OutDataTypeStr=Inherit: Same as input  ParamDataTypeStr=Inherit: Same as input
  Gain4 : Gain  Gain=(1+h)/2  SaturateOnIntegerOverflow=on  OutDataTypeStr=Inherit: Same as input  ParamDataTypeStr=Inherit: Same as input
  Gain6 : Gain  Gain=(1-h)/2  SaturateOnIntegerOverflow=on  OutDataTypeStr=Inherit: Same as input  ParamDataTypeStr=Inherit: Same as input
  Gain9 : Gain  Gain=h  SaturateOnIntegerOverflow=on  OutDataTypeStr=Inherit: Same as input  ParamDataTypeStr=Inherit: Same as input
  Matrix Gain1 : StateSpace  A=[]  B=[]  C=[]  D=K  InitialCondition=0  mask(Matrix Gain){K=Ti'}
      mask prompts: K "Gain matrix:"
      mask help: Matrix Gain.
      mask Help: Multiplies input vector by entered matrix to produce output vector (y=Au).
      mask Display: disp('K')
  Matrix Gain2 : StateSpace  A=[]  B=[]  C=[]  D=K  InitialCondition=0  mask(Matrix Gain){K=Ti}
      mask prompts: K "Gain matrix:"
      mask help: Matrix Gain.
      mask Help: Multiplies input vector by entered matrix to produce output vector (y=Au).
      mask Display: disp('K')
  Subsystem : Subsystem
  Sum1 : Sum  Inputs=-+  InputSameDT=on  SaturateOnIntegerOverflow=on  OutDataTypeStr=Inherit: Same as first input
  Sum3 : Sum  InputSameDT=on  SaturateOnIntegerOverflow=on  OutDataTypeStr=Inherit: Same as first input
  i : Outport  InitialOutput=0  VectorParamsAs1DForOutWhenUnconnected=off
  hist_out : Outport  Port=2  VectorParamsAs1DForOutWhenUnconnected=off
  wires:
  Matrix Gain2/1 -> i/1
  Matrix Gain1/1 -> (1+h)/Z/1
  Gain4/1 -> hist_out/1
  Gain9/1 -> Sum1/1
  Sum3/1 -> Matrix Gain2/1, Gain9/1
  (1+h)/Z/1 -> Sum1/2
  v/1 -> Matrix Gain1/1
  Gain6/1 -> Sum3/1
  hist_in/1 -> Sum3/2
  Subsystem/1(Out1) -> Gain4/1, Gain6/1
  Sum1/1 -> Subsystem/1(In1)

== system simetran/MATE Switch Identifier/inv1 ==
  gate : Inport
  Constant1 : Constant
  Sum3 : Sum  Inputs=-+
  Out1 : Outport
  wires:
  Sum3/1 -> Out1/1
  gate/1 -> Sum3/1
  Constant1/1 -> Sum3/2

== system simetran/MATE_SSE_3Level/Subsystem ==
  g : Inport
  Capacitor : fl_lib/Electrical/Electrical Elements/Capacitor  c=SnubberCapacitance F  r=0 Ohm  g=0 1/Ohm  i_specify=off  i_priority=None  i=0 A  i_nominal_specify=off  i_nominal_value=1  i_nominal_unit=A  v_specify=off  v_priority=None  v=0 V  v_nominal_specify=off  v_nominal_value=1  v_nominal_unit=V  vc_specify=off  vc_priority=High  vc=0 V  vc_nominal_specify=off  vc_nominal_value=1  vc_nominal_unit=V
  Resistor : fl_lib/Electrical/Electrical Elements/Resistor  R=SnubberResistance Ohm  i_specify=off  i_priority=None  i=0 A  i_nominal_specify=off  i_nominal_value=1  i_nominal_unit=A  v_specify=off  v_priority=None  v=0 V  v_nominal_specify=off  v_nominal_value=1  v_nominal_unit=V
  SPST Switch : ee_lib/Switches & Breakers/SPST Switch  R_closed=Ron*2 Ohm  G_open=1e-6 S  Threshold=0.5 V  Width=0 V  model_dynamics=0  t_on=1e-3 s  t_off=1e-3 s  initial_vT=0 V
      settings: InternalSimscapePortConfiguration="{\"Bottom\":[],\"Left\":[{\"id\":\"vT\",\"label\":\"vT\",\"type\":\"input\"},{\"id\":\"p\",\"label\":\"\",\"type\":\"foundation.electrical.electrical\"}],\"Right\":[{\"id\":\"n\",\"label\":\"\",\"type\":\"foundation.electrical.electrical\"}],\"Top\":[]}"
  Simulink-PS Converter : nesl_utility/Simulink-PS Converter  PhysicalDomain=network_engine_domain  SubClassName=ps_input  LeftPortType=input  RightPortType=output  PseudoPeriodic=off  Frequencies=[]  NoiseDistribution=none  NoiseParameters=[]  Unit=1  AffineConversion=off  FilteringAndDerivatives=provide  SimscapeFilterOrder=1  InputFilterTimeConstant=0.001  UdotUserProvided=0
  P : PMIOPort  Side=Left
  N : PMIOPort  Port=2  Side=Right
  wires:
  g/1 -> Simulink-PS Converter/1
  connections:
  SPST Switch/LConn2 -- Capacitor/LConn1 -- P/RConn1
  Simulink-PS Converter/RConn1 -- SPST Switch/LConn1
  SPST Switch/RConn1 -- Resistor/RConn1 -- N/RConn1
  Capacitor/RConn1 -- Resistor/LConn1

== system simetran/MATE_SSE_3Level/Subsystem1 ==
  g : Inport
  Capacitor : fl_lib/Electrical/Electrical Elements/Capacitor  c=SnubberCapacitance F  r=0 Ohm  g=0 1/Ohm  i_specify=off  i_priority=None  i=0 A  i_nominal_specify=off  i_nominal_value=1  i_nominal_unit=A  v_specify=off  v_priority=None  v=0 V  v_nominal_specify=off  v_nominal_value=1  v_nominal_unit=V  vc_specify=off  vc_priority=High  vc=0 V  vc_nominal_specify=off  vc_nominal_value=1  vc_nominal_unit=V
  Resistor : fl_lib/Electrical/Electrical Elements/Resistor  R=SnubberResistance Ohm  i_specify=off  i_priority=None  i=0 A  i_nominal_specify=off  i_nominal_value=1  i_nominal_unit=A  v_specify=off  v_priority=None  v=0 V  v_nominal_specify=off  v_nominal_value=1  v_nominal_unit=V
  SPST Switch : ee_lib/Switches & Breakers/SPST Switch  R_closed=Ron*2 Ohm  G_open=1e-6 S  Threshold=0.5 V  Width=0 V  model_dynamics=0  t_on=1e-3 s  t_off=1e-3 s  initial_vT=0 V
      settings: InternalSimscapePortConfiguration="{\"Bottom\":[],\"Left\":[{\"id\":\"vT\",\"label\":\"vT\",\"type\":\"input\"},{\"id\":\"p\",\"label\":\"\",\"type\":\"foundation.electrical.electrical\"}],\"Right\":[{\"id\":\"n\",\"label\":\"\",\"type\":\"foundation.electrical.electrical\"}],\"Top\":[]}"
  Simulink-PS Converter : nesl_utility/Simulink-PS Converter  PhysicalDomain=network_engine_domain  SubClassName=ps_input  LeftPortType=input  RightPortType=output  PseudoPeriodic=off  Frequencies=[]  NoiseDistribution=none  NoiseParameters=[]  Unit=1  AffineConversion=off  FilteringAndDerivatives=provide  SimscapeFilterOrder=1  InputFilterTimeConstant=0.001  UdotUserProvided=0
  P : PMIOPort  Side=Left
  N : PMIOPort  Port=2  Side=Right
  wires:
  g/1 -> Simulink-PS Converter/1
  connections:
  SPST Switch/LConn2 -- Capacitor/LConn1 -- P/RConn1
  Simulink-PS Converter/RConn1 -- SPST Switch/LConn1
  SPST Switch/RConn1 -- Resistor/RConn1 -- N/RConn1
  Capacitor/RConn1 -- Resistor/LConn1
